simulink model "HLB_MPC"  (R2019b)
settings: Solver=ode1  StartTime=0.0  StopTime=inf  FixedStep=0.02  RelTol=1e-3
settings Model: Creator=IGG2BP  LastModifiedBy=IGG2BP

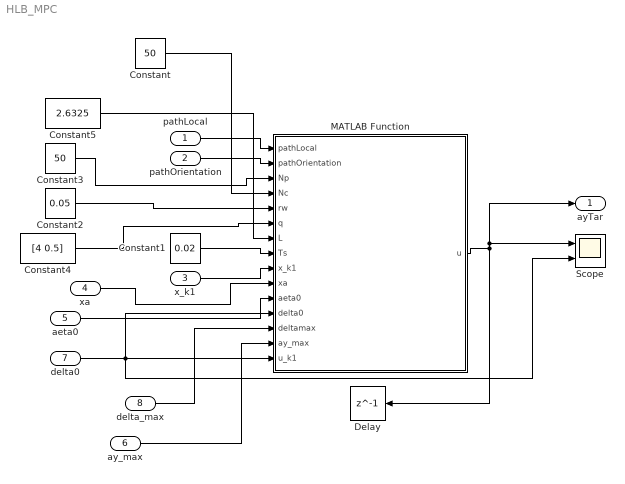
== system HLB_MPC ==
  pathLocal : Inport  PortDimensions=[100,2]
  pathOrientation : Inport  Port=2  PortDimensions=[100,1]
  x_k1 : Inport  Port=3  PortDimensions=[5,1]
  xa : Inport  Port=4  PortDimensions=[7,1]
  aeta0 : Inport  Port=5
  ay_max : Inport  Port=6
  delta0 : Inport  Port=7
  delta_max : Inport  Port=8
  Constant : Constant  Value=50
  Constant1 : Constant  Value=0.02
  Constant2 : Constant  Value=0.05
  Constant3 : Constant  Value=50
  Constant4 : Constant  Value=[4 0.5]
  Constant5 : Constant  Value=2.6325
  Delay : Delay  DelayLength=1  InitialCondition=0
  MATLAB Function : MATLAB Function  TreatAsAtomicUnit=on
  Scope : Scope  NumInputPorts=2
  ayTar : Outport
  wires:
  pathLocal/1 -> MATLAB Function/1(pathLocal)
  pathOrientation/1 -> MATLAB Function/2(pathOrientation)
  x_k1/1 -> MATLAB Function/9(x_k1)
  xa/1 -> MATLAB Function/10(xa)
  aeta0/1 -> MATLAB Function/11(aeta0)
  ay_max/1 -> MATLAB Function/14(ay_max)
  MATLAB Function/1(u) -> ayTar/1, Scope/1, Delay/1
  Constant/1 -> MATLAB Function/4(Nc)
  Constant1/1 -> MATLAB Function/8(Ts)
  Constant2/1 -> MATLAB Function/5(rw)
  Constant3/1 -> MATLAB Function/3(Np)
  Constant4/1 -> MATLAB Function/6(q)
  delta0/1 -> MATLAB Function/12(delta0), Scope/2, MATLAB Function/15(u_k1)
  Constant5/1 -> MATLAB Function/7(L)
  delta_max/1 -> MATLAB Function/13(deltamax)

== matlab function HLB_MPC/MATLAB Function ==
  data: pathLocal input; pathOrientation input; Np input; Nc input; rw input; q input; L input; Ts input; x_k1 input; xa input; aeta0 input; delta0 input; deltamax input; ay_max input; u_k1 input; u output
function u = fcn(pathLocal, pathOrientation, Np, Nc, rw, q, L, Ts,  x_k1, xa, aeta0, delta0, deltamax, ay_max, u_k1)
%% INTRODUCTION
% This function is the core MPC algorithm part.
% created by Gergo Igneczi @ Vehicle Research Center of Szechenyi Istvan
% University

if (x_k1(3) < 3)
    % speed is low, MPC will not work
    u = 0;
else
    dim = 2; % number of outputs
    % producing prediction matrices
    pred_matrix = zeros(min(dim*Np,1000),1);

    x_points = pathLocal(:,1);
    y_points = pathLocal(:,2);

    for i = 1:Np
        %pred_matrix(dim*i-(dim-1),1) = x_points(i);
        pred_matrix(dim*i-(dim-1),1) = y_points(i);
        pred_matrix(dim*i-(dim-2),1) = pathOrientation(i);
    end
    Rs_rk = pred_matrix;

    I = eye(min(Nc,1000));
    %% determining state constraints    

    u_max = ay_max;
    u_min = ay_max;

    %% initializing helper matrices
    M = zeros(min(1000,2*size(u_k1,1)*Nc),min(2*Nc,1000));
    for (i=1:2*size(u_k1,1)*Nc)
        if (i<=(Nc))
            k=1;
            while ((2*k-1)/2 <= i)
                M (i,2*k-1) = 1;
                k = k + 1;
            end
        elseif (i <=(Nc*2))
            k=1;
            while ((2*k-1)/2 <= i-Nc)
                M (i,2*k-1) = -1;
                k = k + 1;
            end
        elseif (i<=(Nc*3))
            k=1;
            while (2*k/2 <= i-size(x_k1,1)*Nc/2)
                M (i,2*k) = 1;
                k = k+1;
            end
        else
            k=1;
            while (2*k/2 <= i-size(x_k1,1)*Nc/2-Nc)
                M (i,2*k) = -1;
                k = k+1;
            end
        end
    end


    %% updating state matrices
    %Ad = [1 0 Ts 0 0; 0 1 0 Ts 0; 0 0 1 0 -Ts/L*x_k1(3)^2*tan(delta0); 0 0 0 1 0; 0 0 0 0 1];
    %Bd = [0 0 0 Ts/L*x_k1(3)^2*1/(cos(delta0))^2 Ts/L*x_k1(3)*1/(cos(delta0))^2]';
    Ad = [1 0 Ts 0 0; 0 1 0 Ts 0; 0 0 1 0 -aeta0*Ts; 0 0 0 1 0;0 0 0 0 1];
    Bd = [0 0 0 Ts Ts/x_k1(3)]';
    Cd = [0 1 0 0 0; 0 0 0 0 1];
    n = size(Ad,1); m = size(Cd,1); k = 1; %size(Bd,2);
    
    %% augmented model
    A = [Ad zeros(n,m); Cd*Ad eye(m,m)];
    B = [Bd; Cd*Bd];
    C = [zeros(m,n) eye(m,m)];
    %% matrix generation
    F = zeros(Np*m,m+n);
    for i=1:Np
        if (m>1)
            F(m*i-(m-1):m*i,1:(m+n))=C*A^i;
        else
            F(i,1:(m+n))=C*A^i;
        end
    end
    S = zeros(m*Np,Nc);
    for i=1:Np
        for j=1:Nc
            if(j>i)
                S(m*i-(m-1):m*i,j)=zeros(m,k);
            else
                S(m*i-(m-1):m*i,j)=C*A^((i-1)-(j-1))*B;
            end
        end
    end

    %% control calculation
    % Unconstrained results
    dU = zeros(min(1000,k*Nc),1);
    %dU = inv(S'*S+rw*I)*(S'*Rs_rk-S'*F*xa);
    R = rw*I;
    Q = zeros(m*Np, m*Np);
    for i=1:Np
        Q(i*numel(q)-(numel(q)-1):i*numel(q),i*numel(q)-(numel(q)-1):i*numel(q)) = diag(q);
    end
    dU = inv(S'*Q*S+R)*S'*Q*(Rs_rk-F*xa);
    
    x = zeros(n,Np);
    x_ = zeros(Np,1);
    y_ = zeros(Np,1);
    u = zeros(Np,1); 
    y= zeros(dim, Np);
    x(:,1) = x_k1;
    u(1) = u_k1;
    speed = x_k1(3);
    theta = 0; 
    vx = speed;
    vy = x_k1(4);
    x_(1) = 0; y_(1) = 0;
    
    for i=2:Np
        if (i < size(dU,1))
            u(i) = u(i-1)+dU(i-1);
        else
            u(i) = u(i-1);
        end
        x(:,i) = Ad*x(:,i-1)+Bd*u(i);
        y(:,i) = Cd*x(:,i);
        % ground truth
        yawRate = u(i) / speed;
        theta = theta + Ts*yawRate;
        ax = -sin(theta)*u(i);
        ay = cos(theta)*u(i);
        vx = vx+Ts*ax;
        vy = vy+Ts*ay;
        x_(i) = x_(i-1)+Ts*vx;
        y_(i) = y_(i-1)+Ts*vy;
    end
    Y = F*xa+S*dU;
    figure(2);
    plot(x(1,:),Y(1:2:end), 'k',x_points,y_points,'b--', x_,y_, 'r');
    grid on; xlim([-5,60]); ylim([-10,10]);

    % Constrained results
    gamma = zeros(min(1000,2*size(u_k1,1)*Nc),1);

    for i=1:2*size(u_k1,1)*Nc
        if (i<=Nc)
            gamma(i,1) = u_max(1)-u_k1(1);
        elseif (i<=2*Nc)
            gamma(i,1) = u_min(1)+u_k1(1);
        end
    end

    if (all(M(:,1:2:end)*dU<=gamma))
        %do nothing
    else
        %Solving Hildreth's QP problem
        E = (S'*S+rw*I)*2;
        F_ = -2*S'*(Rs_rk-F*xa);
        H = E;
        f = F_;
        A_cons = M(:,1:2:end);
        b = gamma;
        eta = x_k1;
        [n1,m1]=size(A_cons);
        eta=-H\f;
        kk=0;
        for i=1:n1
            if (A_cons(i,:)*eta>b(i)) 
                kk=kk+1;
            else
                kk=kk+0;
            end
        end
        if (kk==0) 
            % do nothing 
        else
            P=A_cons*(H\A_cons');
            d=(A_cons*(H\f)+b);
            [n,m]=size(d);
            x_ini=zeros(n,m);
            lambda=x_ini;
            al=10;
            for km=1:38
                %find the elements in the solution vector one by one
                % km could be larger if the Lagranger multiplier has a slow
                % convergence rate.
                lambda_p=lambda;
                for i=1:n
                    w= P(i,:)*lambda-P(i,i)*lambda(i,1);
                    w=w+d(i,1);
                    la=-w/P(i,i);
                    lambda(i,:)=max(0,la);
                end
                al=(lambda-lambda_p)'*(lambda-lambda_p);
                if (al<10e-8)
                    break; 
                end
            end
            dU=-H\f -H\A_cons'*lambda;
        end
    end

    u = u_k1+dU(1);

    %u(1) = min(max(u(1),-ay_max),ay_max);

end


end
